simulink model "LFRefMdl"  (R2023b)
settings: Solver=FixedStepDiscrete  StartTime=0.0  StopTime=inf  FixedStep=Ts  RelTol=1e-3
undefined symbols (not defined in the file or in its folder): Cf, Cr, DataType, default_spacing, hasLag, Iz, lf, lr, m, max_ac, max_steer, min_ac, min_steer, NumEgoStates, posSelector, PredictionHorizon, tau, time_gap, Ts, v0_ego
libraries: mpcsigdimcheck_private x19, mpclib x7, simulink x2, mpcadaslib x1, trackingutilitieslib x1, drivinglib x1
(part 1 of 2)
settings Model: Creator=The MathWorks, Inc.  LastModifiedBy=Luca
settings SolverCC: AlgebraicLoopSolver=TrustRegion
settings DataIOCC: SaveOutput=off  SaveTime=off  ReturnWorkspaceOutputs=off
settings OptimizationCC: DefaultParameterBehavior=Inlined  DefaultUnderspecifiedDataType=single  EnhancedBackFolding=on  PassReuseOutputArgsAs=Individual arguments  ZeroExternalMemoryAtStartup=off  ZeroInternalMemoryAtStartup=off  OptimizeBlockOrder=speed  DifferentSizesBufferReuse=on  OptimizationCustomize=off  EfficientTunableParamExpr=on
settings DebuggingCC: ParameterPrecisionLossMsg=none  ParameterTunabilityLossMsg=error  UnconnectedInputMsg=warning  UnconnectedOutputMsg=warning  UnconnectedLineMsg=warning  PregeneratedLibrarySubsystemCodeDiagnostic=none  ArithmeticOperatorsInVariantConditions=warning
settings HardwareCC: ProdLongLongMode=on
settings ModelReferenceCC: EnableRefExpFcnMdlSchedulingChecks=on
settings SFSimCC: SimUseLocalCustomCode=off  MATLABDynamicMemAlloc=off  CustomCodeUndefinedFunction=UseInterfaceOnly  SimTargetLang=C++
settings RTWCC: Description=Embedded Coder  SystemTargetFile=ert.tlc  TemplateMakefile=ert_default_tmf  GenerateReport=on  RTWUseLocalCustomCode=off  BuildConfiguration=Faster Runs  IncludeHyperlinkInReport=on  LaunchReport=on  TargetLang=C++  GenerateTraceInfo=on  GenerateTraceReport=on  GenerateTraceReportSl=on  GenerateTraceReportSf=on  GenerateTraceReportEml=on  DLArmComputeVersion=19.05
settings CodeAppCC: ForceParamTrailComments=on  IgnoreCustomStorageClasses=off  MaxIdLength=63  OperatorAnnotations=on  SimulinkDataObjDesc=on  SFDataObjDesc=on  CustomSymbolStrFcn=$N$M$F  InsertBlockDesc=on
settings ERTTargetCC: TargetLangStandard=C++03 (ISO)  GenerateSampleERTMain=on  CodeInterfacePackaging=C++ class  InlinedParameterPlacement=NonHierarchical  RootIOFormat=Structure reference  ERTCustomFileTemplate=example_file_process.tlc

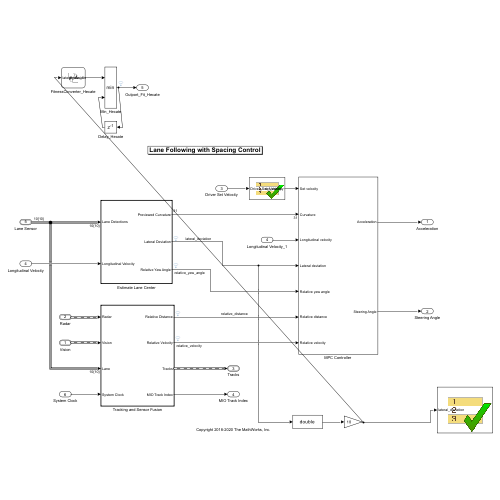
[thumbnail: Simulink's stored preview of the top-level diagram]
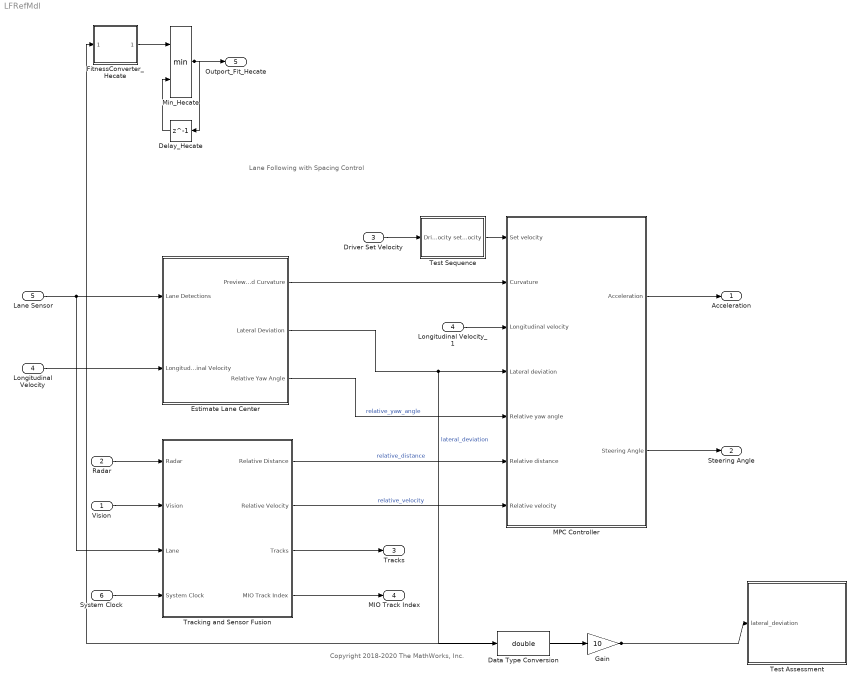
== system LFRefMdl ==
  note: Copyright 2018-2020 The MathWorks, Inc.
  note: Lane Following with Spacing Control
  Vision : Inport  OutDataTypeStr=Bus: BusVision  PortDimensions=[1 1]  BusOutputAsStruct=on
  Radar : Inport  Port=2  OutDataTypeStr=Bus: BusRadar  PortDimensions=[1 1]  BusOutputAsStruct=on
  Driver Set Velocity : Inport  Port=3  OutDataTypeStr=double
  Longitudinal Velocity : Inport  Port=4  OutDataTypeStr=double  Unit=m/s
  Lane Sensor : Inport  Port=5  OutDataTypeStr=Bus: LaneSensor  PortDimensions=[1 1]
  System Clock : Inport  Port=6  OutDataTypeStr=double  PortDimensions=[1 1]
  Data Type Conversion : DataTypeConversion  OutDataTypeStr=double  SaturateOnIntegerOverflow=off  RndMeth=Floor
  Delay_Hecate : Delay  DelayLength=1  InitialCondition=Inf
  Estimate Lane Center : Subsystem  TreatAsAtomicUnit=on  VariantControl=v2
      settings: RTWFileNameOpts=Use function name
  FitnessConverter_Hecate : Stateflow chart  TreatAsAtomicUnit=on
  Gain : Gain  Gain=10
  Longitudinal Velocity_1 : InportShadow  Port=4  OutDataTypeStr=double  Unit=m/s
  "MPC Controller " : Subsystem
  Min_Hecate : MinMax  Inputs=2
  Test Assessment : Test Sequence  TreatAsAtomicUnit=on
  Test Sequence : Test Sequence  TreatAsAtomicUnit=on
  Tracking and Sensor Fusion : Subsystem  TreatAsAtomicUnit=on
      settings: RTWFileNameOpts=Use function name
  Acceleration : Outport  PortDimensions=1  VectorParamsAs1DForOutWhenUnconnected=off
  Steering Angle : Outport  Port=2  PortDimensions=1  VectorParamsAs1DForOutWhenUnconnected=off
  Tracks : Outport  Port=3  OutDataTypeStr=Bus: BusMultiObjectTracker1  PortDimensions=[1 1]  VectorParamsAs1DForOutWhenUnconnected=off  BusOutputAsStruct=on
  MIO Track Index : Outport  Port=4  PortDimensions=1  VectorParamsAs1DForOutWhenUnconnected=off  BusOutputAsStruct=on
  Outport_Fit_Hecate : Outport  Port=5
  wires:
  Longitudinal Velocity/1 -> Estimate Lane Center/2(Longitudinal Velocity)
  Lane Sensor/1 -> Tracking and Sensor Fusion/3(Lane), Estimate Lane Center/1(Lane Detections)
  Vision/1 -> Tracking and Sensor Fusion/2(Vision)
  Radar/1 -> Tracking and Sensor Fusion/1(Radar)
  System Clock/1 -> Tracking and Sensor Fusion/4(System Clock)
  Tracking and Sensor Fusion/3(Tracks) -> Tracks/1
  Tracking and Sensor Fusion/4(MIO Track Index) -> MIO Track Index/1
  Driver Set Velocity/1 -> Test Sequence/1(Driver_Set_Velocity)
  Longitudinal Velocity_1/1 -> "MPC Controller "/3(Longitudinal velocity)
  Estimate Lane Center/1(Previewed Curvature) -> "MPC Controller "/2(Curvature)
  "MPC Controller "/1(Acceleration) -> Acceleration/1
  "MPC Controller "/2(Steering Angle) -> Steering Angle/1
  Estimate Lane Center/2(Lateral Deviation) -> "MPC Controller "/4(Lateral deviation), Data Type Conversion/1  "lateral_deviation"
  Estimate Lane Center/3(Relative Yaw Angle) -> "MPC Controller "/5(Relative yaw angle)  "relative_yaw_angle"
  Tracking and Sensor Fusion/1(Relative Distance) -> "MPC Controller "/6(Relative distance)  "relative_distance"
  Tracking and Sensor Fusion/2(Relative Velocity) -> "MPC Controller "/7(Relative velocity)  "relative_velocity"
  Test Sequence/1(set_velocity) -> "MPC Controller "/1(Set velocity)
  Data Type Conversion/1 -> Gain/1
  Gain/1 -> Test Assessment/1(lateral_deviation), FitnessConverter_Hecate/1(lateral_deviation)
  FitnessConverter_Hecate/1(fitness_1) -> Min_Hecate/1
  Min_Hecate/1 -> Delay_Hecate/1, Outport_Fit_Hecate/1
  Delay_Hecate/1 -> Min_Hecate/2

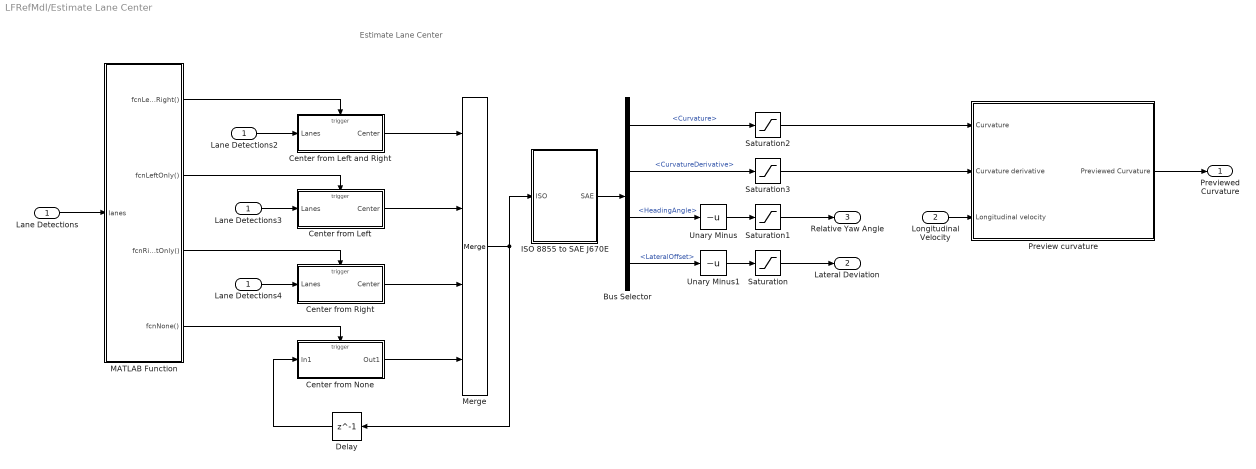
== system LFRefMdl/Estimate Lane Center ==
  note: Estimate Lane Center
  Lane Detections : Inport
  Longitudinal Velocity : Inport  Port=2
  Bus Selector : BusSelector  OutputSignals=Curvature,CurvatureDerivative,HeadingAngle,LateralOffset
  Center from Left : Subsystem  TreatAsAtomicUnit=on
  Center from Left and Right : Subsystem  TreatAsAtomicUnit=on
  Center from None : Subsystem  TreatAsAtomicUnit=on
  Center from Right : Subsystem  TreatAsAtomicUnit=on
  Delay : Delay  DelayLength=1
  ISO 8855 to SAE J670E : Subsystem
  Lane Detections2 : InportShadow
  Lane Detections3 : InportShadow
  Lane Detections4 : InportShadow
  MATLAB Function : MATLAB Function  TreatAsAtomicUnit=on
  Merge : Merge  Inputs=4
  Preview curvature : Subsystem
  Saturation : Saturate  UpperLimit=1.5  LowerLimit=-1.5
  Saturation1 : Saturate  UpperLimit=0.6  LowerLimit=-0.6
  Saturation2 : Saturate  UpperLimit=0.15  LowerLimit=-0.15
  Saturation3 : Saturate  UpperLimit=0.06  LowerLimit=-0.06
  Unary Minus : UnaryMinus
  Unary Minus1 : UnaryMinus
  Previewed Curvature : Outport  VectorParamsAs1DForOutWhenUnconnected=off
  Lateral Deviation : Outport  Port=2  VectorParamsAs1DForOutWhenUnconnected=off
  Relative Yaw Angle : Outport  Port=3  VectorParamsAs1DForOutWhenUnconnected=off
  wires:
  Center from Right/1(Center) -> Merge/3
  Lane Detections3/1 -> Center from Left/1(Lanes)
  Lane Detections4/1 -> Center from Right/1(Lanes)
  MATLAB Function/2(fcnLeftOnly()) -> Center from Left/Trigger
  Center from None/1(Out1) -> Merge/4
  MATLAB Function/1(fcnLeftAndRight()) -> Center from Left and Right/Trigger
  Delay/1 -> Center from None/1(In1)
  Center from Left and Right/1(Center) -> Merge/1
  Lane Detections/1 -> MATLAB Function/1(lanes)
  Lane Detections2/1 -> Center from Left and Right/1(Lanes)
  MATLAB Function/3(fcnRightOnly()) -> Center from Right/Trigger
  MATLAB Function/4(fcnNone()) -> Center from None/Trigger
  Center from Left/1(Center) -> Merge/2
  Merge/1 -> ISO 8855 to SAE J670E/1(ISO), Delay/1
  Saturation3/1 -> Preview curvature/2(Curvature derivative)
  Saturation2/1 -> Preview curvature/1(Curvature)
  Saturation1/1 -> Relative Yaw Angle/1
  Saturation/1 -> Lateral Deviation/1
  Unary Minus/1 -> Saturation1/1
  Preview curvature/1(Previewed Curvature) -> Previewed Curvature/1
  Longitudinal Velocity/1 -> Preview curvature/3(Longitudinal velocity)
  Bus Selector/2 -> Saturation3/1  "<CurvatureDerivative>"
  Bus Selector/1 -> Saturation2/1  "<Curvature>"
  Unary Minus1/1 -> Saturation/1
  Bus Selector/4 -> Unary Minus1/1  "<LateralOffset>"
  Bus Selector/3 -> Unary Minus/1  "<HeadingAngle>"
  ISO 8855 to SAE J670E/1(SAE) -> Bus Selector/1

== system LFRefMdl/MPC Controller  ==
  Set velocity : Inport
  Curvature : Inport  Port=2
  Longitudinal velocity : Inport  Port=3
  Lateral deviation : Inport  Port=4
  Relative yaw angle : Inport  Port=5
  Relative distance : Inport  Port=6
  Relative velocity : Inport  Port=7
  Constant : Constant  Value=time_gap
  Constant1 : Constant  Value=200
  Constant2 : Constant  Value=0
  Path Following Control System : Subsystem  AncestorBlock=mpcadaslib/Path Following Control System  TreatAsAtomicUnit=on  VariantControl=Variant2  mask(Path following control (PFC) system){ModelType=Use vehicle parameters, VehicleMass=m, VehicleYawInertia=Iz, LengthToFront=lf, LengthToRear=lr, FrontTireStiffness=Cf, RearTireStiffness=Cr, AccelTimeConstant=tau, EgoModelMatrixA=[-2,zeros(1,3);1,zeros(1,3);zeros(1,2),-4.4021,-12.4603;zeros(1,2),1.3913,-5.1868], EgoModelMatrixB=[2,zeros(1,3);zeros(1,2),24.1270,15.8609]', EgoModelMatrixC=[zeros(3,1),eye(3)], InitialLongVel=v0_ego, TransportLag=Ts, spaceCtrl=on, DefaultSpacing=default_spacing, MinSteering=min_steer, umin_ext=off, MaxSteering=max_steer, umax_ext=off, MinAcceleration=min_ac, amin_ext=off, MaxAcceleration=max_ac, amax_ext=off, Ts=Ts, PredictionHorizon=PredictionHorizon, ControlHorizon=2, LongWeight=0.1, LateralWeight=1, AccelRateWeight=0.1, SteerRateWeight=0.1, suboptimal=off, maxiter=10, datatypeopt=double, optmode=off, trackmode=off}
      mask prompts: VehicleMass "MPC:adasblocks:promptPFCVehicleMass"; VehicleYawInertia "MPC:adasblocks:promptPFCVehicleInertia"; LengthToFront "MPC:adasblocks:promptPFCVehicleLengthToFront"; LengthToRear "MPC:adasblocks:promptPFCVehicleLengthToRear"; FrontTireStiffness "MPC:adasblocks:promptPFCVehicleFrontStiffness"; RearTireStiffness "MPC:adasblocks:promptPFCVehicleRearStiffness"; AccelTimeConstant "MPC:adasblocks:promptPFCVehicleTimeConstant"; EgoModelMatrixA "MPC:adasblocks:promptPFCMatrixA"; EgoModelMatrixB "MPC:adasblocks:promptPFCMatrixB"; EgoModelMatrixC "MPC:adasblocks:promptPFCMatrixC"; InitialLongVel "MPC:adasblocks:promptPFCInitialLongitudinalVelocity"; TransportLag "MPC:adasblocks:promptPFCTransportLag"; spaceCtrl "MPC:adasblocks:promptPFCSpacingControl"; DefaultSpacing "MPC:adasblocks:promptPFCDefaultSpacing"; MinSteering "MPC:adasblocks:promptPFCMinSteering"; umin_ext "MPC:adasblocks:promptPFCUseExternalSource"; MaxSteering "MPC:adasblocks:promptPFCMaxSteering"; umax_ext "MPC:adasblocks:promptPFCUseExternalSource"; MinAcceleration "MPC:adasblocks:promptPFCMinAcceleration"; amin_ext "MPC:adasblocks:promptPFCUseExternalSource"; MaxAcceleration "MPC:adasblocks:promptPFCMaxAcceleration"; amax_ext "MPC:adasblocks:promptPFCUseExternalSource"; Ts "MPC:adasblocks:promptPFCSampleTime"; PredictionHorizon "MPC:adasblocks:promptPFCPredictionSteps"; ControlHorizon "MPC:adasblocks:promptPFCControlHorizon"; LongWeight "MPC:adasblocks:promptPFCLongWeight"; LateralWeight "MPC:adasblocks:promptPFCLateralWeight"; AccelRateWeight "MPC:adasblocks:promptPFCAccelRateWeight"; SteerRateWeight "MPC:adasblocks:promptPFCSteerRateWeight"; suboptimal "MPC:adasblocks:promptPFCUseSubOptimal"; maxiter "MPC:adasblocks:promptPFCMaxIter"; datatypeopt "MPC:adasblocks:promptPFCDataType"; optmode "MPC:adasblocks:promptPFCMPCOptimize"; trackmode "MPC:adasblocks:promptPFCSmoothTransition"
      mask help: MPC:adasblocks:pfcMaskDescription
      mask init:
      | [mpcobj,hasSpacingCtrl,UseExternalModel,DataType,NumEgoStates,hasLag] = ...
      |     pfcblock_MaskInitFcn(gcb,EgoModelMatrixA,EgoModelMatrixB,EgoModelMatrixC,...
      |     MaxSteering,MinSteering,...
      |     MaxAcceleration,MinAcceleration,...
      |     InitialLongVel,DefaultSpacing,...
      |     PredictionHorizon,ControlHorizon,Ts,maxiter,AccelRateWeight,SteerRateWeight,LongWeight,LateralWeight,...
      |     VehicleMass,VehicleYawInertia,LengthToFront,LengthToRear,FrontTireStiffness,RearTireStiffness,TransportLag,AccelTimeConstant);
      settings: RTWFileNameOpts=Use function name
      mask Help: eval('mpcCSHelp(''mpcBlockPFC'')');
      mask TypeOptions ModelType: MPC:adasblocks:promptPFCUseVehicleParameters | MPC:adasblocks:promptPFCUseVehicleModel
      mask Callback ModelType: pfcblock_callbackModelType(gcb);
      mask Callback spaceCtrl: pfcblock_callbackSpacingCtrl(gcb);
      mask Callback umin_ext: adasblocks_utilUseExternal(gcb,'MinSteering','umin_ext');
      mask Callback umax_ext: adasblocks_utilUseExternal(gcb,'MaxSteering','umax_ext');
      mask Callback amin_ext: adasblocks_utilUseExternal(gcb,'MinAcceleration','amin_ext');
      mask Callback amax_ext: adasblocks_utilUseExternal(gcb,'MaxAcceleration','amax_ext');
      mask Callback suboptimal: adasblocks_callbackUsesuboptimal(gcb);
      mask TypeOptions datatypeopt: double | single
      mask DialogControl DescTextVar Tooltip: MPC:adasblocks:ttipPFCMaskDescription
      mask DialogControl Container4 Prompt: MPC:adasblocks:promptPFCTabParameters
      mask DialogControl Container11 Prompt: MPC:adasblocks:promptPFCEgoVehicle
      mask DialogControl Control4 Prompt: MPC:adasblocks:promptPFCLinearModel
      mask DialogControl ModelType Tooltip: MPC:adasblocks:ttipPFCModelDynamics
      mask DialogControl UseParam Prompt: MPC:adasblocks:promptPFCSpecifyVehicleParameters
      mask DialogControl VehicleMass Prompt: Total mass (kg)
      mask DialogControl VehicleMass Tooltip: MPC:adasblocks:ttipPFCVehicleMass
      mask DialogControl VehicleYawInertia Prompt: Yaw moment of inertia (kgm^2)
      mask DialogControl VehicleYawInertia Tooltip: MPC:adasblocks:ttipPFCVehicleInertia
      mask DialogControl LengthToFront Prompt: Longitudinal distance from center of gravity to front tires (m)
      mask DialogControl LengthToFront Tooltip: MPC:adasblocks:ttipPFCVehicleLengthToFront
      mask DialogControl LengthToRear Prompt: Longitudinal distance from center of gravity to rear tires (m)
      mask DialogControl LengthToRear Tooltip: MPC:adasblocks:ttipPFCVehicleLengthToRear
      mask DialogControl FrontTireStiffness Prompt: Cornering stiffness of front tires (N/rad)
      mask DialogControl FrontTireStiffness Tooltip: MPC:adasblocks:ttipPFCVehicleFrontStiffness
      mask DialogControl RearTireStiffness Prompt: Cornering stiffness of rear tires (N/rad)
      mask DialogControl RearTireStiffness Tooltip: MPC:adasblocks:ttipPFCVehicleRearStiffness
      mask DialogControl AccelTimeConstant Prompt: Longitudinal acceleration tracking time constant (s)
      mask DialogControl AccelTimeConstant Tooltip: MPC:adasblocks:ttipPFCAccelTimeConstant
      mask DialogControl UseModel Prompt: MPC:adasblocks:promptPFCSpecifyVehicleModel
      mask DialogControl EgoModelMatrixA Prompt: A
      mask DialogControl EgoModelMatrixA Tooltip: MPC:adasblocks:ttipPFCEgoModelMatrixA
      mask DialogControl EgoModelMatrixB Prompt: B
      mask DialogControl EgoModelMatrixB Tooltip: MPC:adasblocks:ttipPFCEgoModelMatrixB
      mask DialogControl EgoModelMatrixC Prompt: C
      mask DialogControl EgoModelMatrixC Tooltip: MPC:adasblocks:ttipPFCEgoModelMatrixC
      mask DialogControl InitialLongVel Prompt: Initial longitudinal velocity (m/s)
      mask DialogControl InitialLongVel Tooltip: MPC:adasblocks:ttipPFCInitialLongVelocity
      mask DialogControl TransportLag Prompt: Transport lag between model inputs and outputs (s)
      mask DialogControl TransportLag Tooltip: MPC:adasblocks:ttipPFCTransportLag
      mask DialogControl Container25 Prompt: MPC:adasblocks:promptPFCSpacingCtrl
      mask DialogControl spaceCtrl Prompt: Maintain safe distance between lead vehicle and ego vehicle
      mask DialogControl spaceCtrl Tooltip: MPC:adasblocks:ttipPFCEnableSpacingCtrl
      mask DialogControl DefaultSpacing Prompt: Default spacing (m)
      mask DialogControl DefaultSpacing Tooltip: MPC:adasblocks:ttipPFCDefaultSpacing
      mask DialogControl Container21 Prompt: MPC:adasblocks:promptPFCTabController
      mask DialogControl Container12 Prompt: MPC:adasblocks:promptPFCConstraints
      mask DialogControl MinSteering Prompt: Minimum steering angle (rad)
      mask DialogControl MinSteering Tooltip: MPC:adasblocks:ttipPFCMinSteering
      mask DialogControl umin_ext Prompt: Use external source
      mask DialogControl MaxSteering Prompt: Maximum steering angle (rad)
      mask DialogControl MaxSteering Tooltip: MPC:adasblocks:ttipPFCMaxSteering
      mask DialogControl umax_ext Prompt: Use external source
      mask DialogControl MinAcceleration Prompt: Minimum longitudinal acceleration (m/s^2)
      mask DialogControl MinAcceleration Tooltip: MPC:adasblocks:ttipPFCMaxDeceleration
      mask DialogControl amin_ext Prompt: Use external source
      mask DialogControl MaxAcceleration Prompt: Maximum longitudinal acceleration (m/s^2)
      mask DialogControl MaxAcceleration Tooltip: MPC:adasblocks:ttipPFCMaxAcceleration
      mask DialogControl amax_ext Prompt: Use external source
      mask DialogControl Container15 Prompt: MPC:adasblocks:promptPFCMPCSettings
      mask DialogControl Ts Prompt: Sample time (s)
      mask DialogControl Ts Tooltip: MPC:adasblocks:ttipPFCSampleTime
      mask DialogControl PredictionHorizon Prompt: Prediction horizon (steps)
      mask DialogControl PredictionHorizon Tooltip: MPC:adasblocks:ttipPFCPredictionSteps
      mask DialogControl ControlHorizon Prompt: Control horizon (steps)
      mask DialogControl ControlHorizon Tooltip: MPC:adasblocks:ttipPFCControlHorizon
      mask DialogControl Container18 Prompt: MPC:adasblocks:promptPFCWeight
      mask DialogControl LongWeight Prompt: Weight on velocity tracking
      mask DialogControl LongWeight Tooltip: MPC:adasblocks:ttipPFCLongWeight
      mask DialogControl LateralWeight Prompt: Weight on lateral error
      mask DialogControl LateralWeight Tooltip: MPC:adasblocks:ttipPFCLateralWeight
      mask DialogControl AccelRateWeight Prompt: Weight on change of longitudinal acceleration
      mask DialogControl AccelRateWeight Tooltip: MPC:adasblocks:ttipPFCAccelRateWeight
      mask DialogControl SteerRateWeight Prompt: Weight on change of steering angle
      mask DialogControl SteerRateWeight Tooltip: MPC:adasblocks:ttipPFCSteerRateWeight
      mask DialogControl Container6 Prompt: MPC:adasblocks:promptPFCTabBlock
      mask DialogControl Container7 Prompt: MPC:adasblocks:promptPFCOptimization
      mask DialogControl suboptimal Prompt: Use suboptimal solution
      mask DialogControl suboptimal Tooltip: MPC:adasblocks:ttipPFCUseSubOptimal
      mask DialogControl maxiter Prompt: Maximum iteration number
      mask DialogControl maxiter Tooltip: MPC:adasblocks:ttipPFCMaxIter
      mask DialogControl datatypeopt Prompt: Data Type
      mask DialogControl datatypeopt Tooltip: MPC:adasblocks:ttipPFCDataType
      mask DialogControl Container9 Prompt: MPC:adasblocks:promptPFCBlockOptions
      mask DialogControl optmode Prompt: Use external signal to enable or disable optimization
      mask DialogControl optmode Tooltip: MPC:adasblocks:ttipPFCMPCOptimize
      mask DialogControl trackmode Prompt: Use external control signal for bumpless transfer between PFC and other controllers
      mask DialogControl trackmode Tooltip: MPC:adasblocks:ttipPFCSmoothTransition
      mask DialogControl Container10 Prompt: MPC:adasblocks:promptPFCCustomizeText
      mask DialogControl Control2 Prompt: MPC:adasblocks:promptPFCCreateSystemTextMore
      mask DialogControl Control3 Prompt: MPC:adasblocks:promptPFCCreateSysBtn
      mask DialogControl Control3 Tooltip: MPC:adasblocks:ttipPFCCreateSysBtn
      mask DialogControl Control3 Callback: pfcblock_callbackCreateSubsystemButton(gcb);
  Switch1 : Switch  Criteria=u2 > Threshold  Threshold=1000  SaturateOnIntegerOverflow=off  InputSameDT=off
  Switch2 : Switch  Criteria=u2 > Threshold  Threshold=1000  SaturateOnIntegerOverflow=off  InputSameDT=off
  Acceleration : Outport  VectorParamsAs1DForOutWhenUnconnected=off
  Steering Angle : Outport  Port=2  VectorParamsAs1DForOutWhenUnconnected=off
  wires:
  Path Following Control System/1(Longitudinal acceleration) -> Acceleration/1
  Path Following Control System/2(Steering angle) -> Steering Angle/1
  Set velocity/1 -> Path Following Control System/1(Set velocity)
  Curvature/1 -> Path Following Control System/6(Curvature)
  Longitudinal velocity/1 -> Path Following Control System/5(Longitudinal velocity)
  Lateral deviation/1 -> Path Following Control System/7(Lateral deviation)
  Relative yaw angle/1 -> Path Following Control System/8(Relative yaw angle)
  Relative distance/1 -> Switch2/2, Switch1/3, Switch1/2
  Constant1/1 -> Switch1/1
  Relative velocity/1 -> Switch2/3
  Constant2/1 -> Switch2/1
  Constant/1 -> Path Following Control System/2(Time gap)
  Switch1/1 -> Path Following Control System/3(Relative distance)
  Switch2/1 -> Path Following Control System/4(Relative velocity)

== system LFRefMdl/Tracking and Sensor Fusion ==
  note: Tracking and Sensor Fusion
  note: Sensor Fusion
  Radar : Inport  OutDataTypeStr=Bus: BusRadar  PortDimensions=[1 1]  BusOutputAsStruct=on
  Vision : Inport  Port=2  OutDataTypeStr=Bus: BusVision  PortDimensions=[1 1]  BusOutputAsStruct=on
  Lane : Inport  Port=3  OutDataTypeStr=Bus: LaneSensor  BusOutputAsStruct=on
  System Clock : Inport  Port=4  OutDataTypeStr=double  PortDimensions=[1 1]
  Detection Concatenation1 : trackingutilitieslib/Detection Concatenation  NumInputs=2  BusNameSource=Auto  BusName=BusDetectionConcatenation1  SimulateUsing=Interpreted execution
  Find Lead Car : MATLAB Function  TreatAsAtomicUnit=on
  Multi-Object Tracker : drivinglib/Multi-Object Tracker  TrackerIndex=uint32( 0 )  FilterInitializationFcn=initcvekf  AssignmentThreshold=assigThresh  ConfirmationThreshold=[ 2, 3 ]  DeletionThreshold=[ 5, 5 ]  MaxNumTracks=numTracks  MaxNumSensors=numSensors  OOSMHandling=Terminate  StateParametersSimulink=struct  HasStateParametersInput=off  TimeInputSource=Input port  HasCostMatrixInput=off  HasDetectableTrackIDsInput=off  BusNameSource=Property  BusName=BusMultiObjectTracker1  TentativeTracksOutputPort=off  AllTracksOutputPort=off  SimulateUsing=Interpreted execution
  Position Selector : Constant  Value=posSelector
  Relative Distance : Outport  VectorParamsAs1DForOutWhenUnconnected=off
  Relative Velocity : Outport  Port=2  VectorParamsAs1DForOutWhenUnconnected=off
  Tracks : Outport  Port=3  OutDataTypeStr=Bus:BusMultiObjectTracker1  PortDimensions=[1 1]  VectorParamsAs1DForOutWhenUnconnected=off  BusOutputAsStruct=on
  MIO Track Index : Outport  Port=4  VectorParamsAs1DForOutWhenUnconnected=off
  wires:
  Find Lead Car/2(vx) -> Relative Velocity/1
  Find Lead Car/3(mioTrackIndex) -> MIO Track Index/1
  Find Lead Car/1(x) -> Relative Distance/1
  Position Selector/1 -> Find Lead Car/3(positionSelector)
  Lane/1 -> Find Lead Car/2(lane)
  Detection Concatenation1/1 -> Multi-Object Tracker/1
  Multi-Object Tracker/1 -> Find Lead Car/1(confirmedTracks), Tracks/1
  System Clock/1 -> Multi-Object Tracker/2
  Vision/1 -> Detection Concatenation1/1
  Radar/1 -> Detection Concatenation1/2

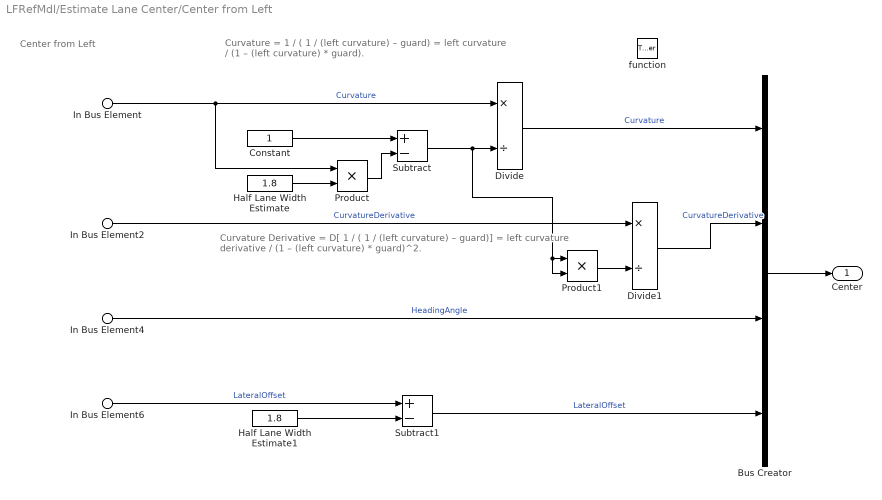
== system LFRefMdl/Estimate Lane Center/Center from Left ==
  note: Curvature Derivative
      | = D[ 1 / ( 1 / (left curvature) – guard)]
      | = left curvature derivative / (1 – (left curvature) * guard)^2.
  note: Center from Left
  note: Curvature
      | = 1 / ( 1 / (left curvature) – guard)
      | = left curvature / (1 – (left curvature) * guard).
  In Bus Element : Inport  PortName=Lanes  Element=Left.Curvature
  In Bus Element2 : Inport  PortName=Lanes  Element=Left.CurvatureDerivative
  In Bus Element4 : Inport  PortName=Lanes  Element=Left.HeadingAngle
  In Bus Element6 : Inport  PortName=Lanes  Element=Left.LateralOffset
  function : TriggerPort  TriggerType=function-call  VariantControl=Variant
  Bus Creator : BusCreator  Inputs=4
  Constant : Constant  OutDataTypeStr=Inherit: Inherit via back propagation
  Divide : Product  Inputs=*/
  Divide1 : Product  Inputs=*/
  Half Lane Width Estimate : Constant  Value=1.8  OutDataTypeStr=Inherit: Inherit via back propagation
  Half Lane Width Estimate1 : Constant  Value=1.8  OutDataTypeStr=Inherit: Inherit via back propagation
  Product : Product
  Product1 : Product
  Subtract : Sum  Inputs=+-
  Subtract1 : Sum  Inputs=+-
  Center : Outport  VectorParamsAs1DForOutWhenUnconnected=off
  wires:
  Product/1 -> Subtract/2
  Half Lane Width Estimate1/1 -> Subtract1/2
  In Bus Element6/1 -> Subtract1/1  "LateralOffset"
  Product1/1 -> Divide1/2
  In Bus Element2/1 -> Divide1/1  "CurvatureDerivative"
  Constant/1 -> Subtract/1
  Half Lane Width Estimate/1 -> Product/2
  Subtract/1 -> Divide/2, Product1/1, Product1/2
  In Bus Element/1 -> Divide/1, Product/1  "Curvature"
  Subtract1/1 -> Bus Creator/4  "LateralOffset"
  In Bus Element4/1 -> Bus Creator/3  "HeadingAngle"
  Divide/1 -> Bus Creator/1  "Curvature"
  Divide1/1 -> Bus Creator/2  "CurvatureDerivative"
  Bus Creator/1 -> Center/1

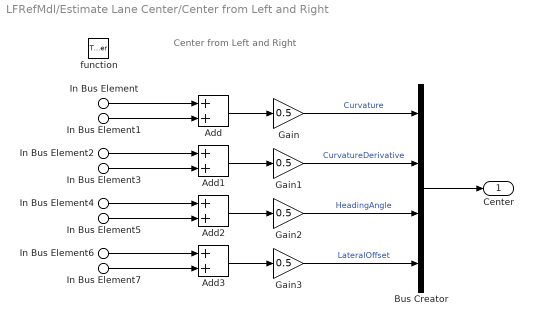
== system LFRefMdl/Estimate Lane Center/Center from Left and Right ==
  note: Center from Left and Right
  In Bus Element : Inport  PortName=Lanes  Element=Left.Curvature
  In Bus Element2 : Inport  PortName=Lanes  Element=Left.CurvatureDerivative
  In Bus Element4 : Inport  PortName=Lanes  Element=Left.HeadingAngle
  In Bus Element6 : Inport  PortName=Lanes  Element=Left.LateralOffset
  In Bus Element1 : Inport  PortName=Lanes  Element=Right.Curvature
  In Bus Element3 : Inport  PortName=Lanes  Element=Right.CurvatureDerivative
  In Bus Element5 : Inport  PortName=Lanes  Element=Right.HeadingAngle
  In Bus Element7 : Inport  PortName=Lanes  Element=Right.LateralOffset
  function : TriggerPort  TriggerType=function-call  VariantControl=Variant
  Add{,1..3} (4 alike) : Sum
  Bus Creator : BusCreator  Inputs=4
  Gain{,1..3} (4 alike) : Gain  Gain=0.5
  Center : Outport  VectorParamsAs1DForOutWhenUnconnected=off
  wires:
  In Bus Element6/1 -> Add3/1
  In Bus Element7/1 -> Add3/2
  In Bus Element5/1 -> Add2/2
  In Bus Element4/1 -> Add2/1
  In Bus Element3/1 -> Add1/2
  In Bus Element2/1 -> Add1/1
  In Bus Element1/1 -> Add/2
  In Bus Element/1 -> Add/1
  Bus Creator/1 -> Center/1
  Gain3/1 -> Bus Creator/4  "LateralOffset"
  Add3/1 -> Gain3/1
  Gain2/1 -> Bus Creator/3  "HeadingAngle"
  Add2/1 -> Gain2/1
  Gain1/1 -> Bus Creator/2  "CurvatureDerivative"
  Add1/1 -> Gain1/1
  Gain/1 -> Bus Creator/1  "Curvature"
  Add/1 -> Gain/1

== system LFRefMdl/Estimate Lane Center/Center from None ==
  In1 : Inport
  function : TriggerPort  TriggerType=function-call  VariantControl=Variant
  Out1 : Outport  VectorParamsAs1DForOutWhenUnconnected=off
  wires:
  In1/1 -> Out1/1

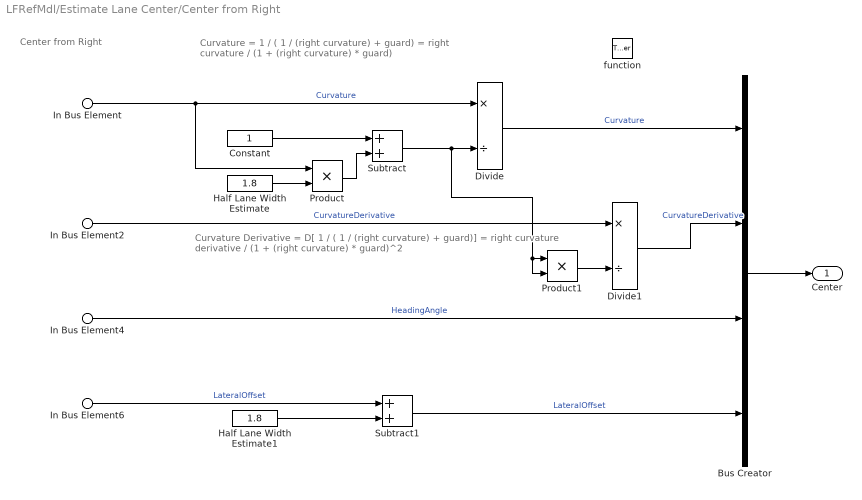
== system LFRefMdl/Estimate Lane Center/Center from Right ==
  note: Curvature Derivative
      | = D[ 1 / ( 1 / (right curvature) + guard)]
      | = right curvature derivative / (1 + (right curvature) * guard)^2
  note: Curvature
      | = 1 / ( 1 / (right curvature) + guard)
      | = right curvature / (1 + (right curvature) * guard)
  note: Center from Right
  In Bus Element : Inport  PortName=Lanes  Element=Right.Curvature
  In Bus Element2 : Inport  PortName=Lanes  Element=Right.CurvatureDerivative
  In Bus Element4 : Inport  PortName=Lanes  Element=Right.HeadingAngle
  In Bus Element6 : Inport  PortName=Lanes  Element=Right.LateralOffset
  function : TriggerPort  TriggerType=function-call  VariantControl=Variant
  Bus Creator : BusCreator  Inputs=4
  Constant : Constant  OutDataTypeStr=Inherit: Inherit via back propagation
  Divide : Product  Inputs=*/
  Divide1 : Product  Inputs=*/
  Half Lane Width Estimate : Constant  Value=1.8  OutDataTypeStr=Inherit: Inherit via back propagation
  Half Lane Width Estimate1 : Constant  Value=1.8  OutDataTypeStr=Inherit: Inherit via back propagation
  Product : Product
  Product1 : Product
  Subtract : Sum
  Subtract1 : Sum
  Center : Outport  VectorParamsAs1DForOutWhenUnconnected=off
  wires:
  Half Lane Width Estimate/1 -> Product/2
  Product/1 -> Subtract/2
  Constant/1 -> Subtract/1
  Subtract/1 -> Divide/2, Product1/1, Product1/2
  In Bus Element/1 -> Divide/1, Product/1  "Curvature"
  Bus Creator/1 -> Center/1
  Subtract1/1 -> Bus Creator/4  "LateralOffset"
  Divide/1 -> Bus Creator/1  "Curvature"
  In Bus Element6/1 -> Subtract1/1  "LateralOffset"
  Half Lane Width Estimate1/1 -> Subtract1/2
  In Bus Element4/1 -> Bus Creator/3  "HeadingAngle"
  Product1/1 -> Divide1/2
  Divide1/1 -> Bus Creator/2  "CurvatureDerivative"
  In Bus Element2/1 -> Divide1/1  "CurvatureDerivative"

== system LFRefMdl/Estimate Lane Center/ISO 8855 to SAE J670E ==
  note: positive Y is to the left in ISO 8855
      | positive Y is to the right in SAE J670E
  note: ISO 8855 to SAE J670E
  ISO : Inport
  Bus Creator : BusCreator  Inputs=4
  Bus Selector : BusSelector  OutputSignals=CurvatureDerivative,Curvature,HeadingAngle,LateralOffset
  Signal Specification : SignalSpecification  Unit=1/m^2
  Signal Specification1 : SignalSpecification  Unit=1/m
  Signal Specification2 : SignalSpecification  Unit=rad
  Signal Specification3 : SignalSpecification  Unit=m
  Unary Minus{,1..3} (4 alike) : UnaryMinus
  SAE : Outport  VectorParamsAs1DForOutWhenUnconnected=off
  wires:
  ISO/1 -> Bus Selector/1
  Bus Selector/2 -> Unary Minus/1  "<Curvature>"
  Bus Selector/1 -> Unary Minus1/1  "<CurvatureDerivative>"
  Bus Selector/3 -> Unary Minus2/1  "<HeadingAngle>"
  Bus Selector/4 -> Unary Minus3/1  "<LateralOffset>"
  Bus Creator/1 -> SAE/1
  Signal Specification/1 -> Bus Creator/2  "Curvature"
  Unary Minus1/1 -> Signal Specification1/1
  Unary Minus2/1 -> Signal Specification2/1
  Unary Minus3/1 -> Signal Specification3/1
  Unary Minus/1 -> Signal Specification/1
  Signal Specification1/1 -> Bus Creator/1  "CurvatureDerivative"
  Signal Specification2/1 -> Bus Creator/3  "HeadingAngle"
  Signal Specification3/1 -> Bus Creator/4  "LateralOffset"

== system LFRefMdl/Estimate Lane Center/Preview curvature ==
  Curvature : Inport
  Curvature derivative : Inport  Port=2
  Longitudinal velocity : Inport  Port=3
  Gain : Gain  Gain=[0:Ts:PredictionHorizon*Ts]'
  Gain1 : Gain
  Product : Product
  Sum : Sum
  Previewed Curvature : Outport  VectorParamsAs1DForOutWhenUnconnected=off
  wires:
  Sum/1 -> Previewed Curvature/1
  Curvature/1 -> Gain1/1
  Gain/1 -> Sum/2
  Product/1 -> Gain/1
  Longitudinal velocity/1 -> Product/2
  Curvature derivative/1 -> Product/1
  Gain1/1 -> Sum/1

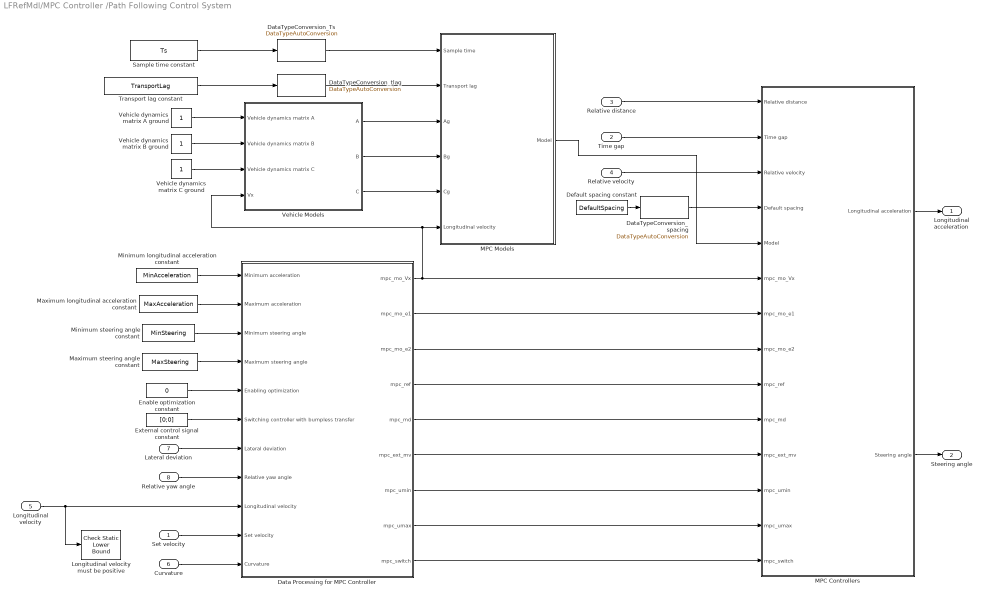
== system LFRefMdl/MPC Controller /Path Following Control System ==
  Set velocity : Inport
  Time gap : Inport  Port=2
  Relative distance : Inport  Port=3
  Relative velocity : Inport  Port=4
  Longitudinal velocity : Inport  Port=5
  Curvature : Inport  Port=6
  Lateral deviation : Inport  Port=7
  Relative yaw angle : Inport  Port=8
  Data Processing for MPC Controller : Subsystem
  DataTypeConversion_Ts : mpcsigdimcheck_private/DataTypeAutoConversion  datatypestr=DataType
  DataTypeConversion_spacing : mpcsigdimcheck_private/DataTypeAutoConversion  datatypestr=DataType
  DataTypeConversion_tlag : mpcsigdimcheck_private/DataTypeAutoConversion  datatypestr=DataType
  Default spacing constant : Constant  Value=DefaultSpacing
  Enable optimization constant : Constant  Value=0
  External control signal constant : Constant  Value=[0;0]  VectorParams1D=off
  Longitudinal velocity must be positive : simulink/Model Verification/Check Static  Lower Bound  Description=0 < u  min=0  min_included=off  enabled=on  stopWhenAssertionFail=off  export=off  icon=graphic
  MPC Controllers : Subsystem  Variant=on  VariantControlMode=label  VariantControl=Variant1  LabelModeActiveChoice=pathFollowingHasSpacingCtrl
  MPC Models : Subsystem  Variant=on  VariantControlMode=label  VariantControl=Variant1  LabelModeActiveChoice=pathFollowingHasSpacingCtrl
  Maximum longitudinal acceleration constant : Constant  Value=MaxAcceleration
  Maximum steering angle constant : Constant  Value=MaxSteering
  Minimum longitudinal acceleration constant : Constant  Value=MinAcceleration
  Minimum steering angle constant : Constant  Value=MinSteering
  Sample time constant : Constant  Value=Ts
  Transport lag constant : Constant  Value=TransportLag
  Vehicle Models : Subsystem  Variant=on  VariantControlMode=label  VariantControl=Variant1  LabelModeActiveChoice=useVehicleParameters
  Vehicle dynamics matrix A ground : Constant
  Vehicle dynamics matrix B ground : Constant
  Vehicle dynamics matrix C ground : Constant
  Longitudinal acceleration : Outport  PortDimensions=1  VectorParamsAs1DForOutWhenUnconnected=off
  Steering angle : Outport  Port=2  VectorParamsAs1DForOutWhenUnconnected=off
  wires:
  DataTypeConversion_spacing/1 -> MPC Controllers/4("Default spacing ")
  DataTypeConversion_tlag/1 -> MPC Models/2(Transport lag)
  DataTypeConversion_Ts/1 -> MPC Models/1(Sample time)
  Vehicle dynamics matrix B ground/1 -> Vehicle Models/2(Vehicle dynamics matrix B)
  Vehicle dynamics matrix C ground/1 -> Vehicle Models/3(Vehicle dynamics matrix C)
  Vehicle dynamics matrix A ground/1 -> Vehicle Models/1(Vehicle dynamics matrix A)
  Sample time constant/1 -> DataTypeConversion_Ts/1
  Transport lag constant/1 -> DataTypeConversion_tlag/1
  Vehicle Models/3(" C") -> MPC Models/5(Cg)
  Vehicle Models/2(" B") -> MPC Models/4(Bg)
  Vehicle Models/1(" A") -> MPC Models/3(Ag)
  Minimum steering angle constant/1 -> Data Processing for MPC Controller/3(Minimum steering angle)
  Minimum longitudinal acceleration constant/1 -> Data Processing for MPC Controller/1(Minimum acceleration)
  External control signal constant/1 -> Data Processing for MPC Controller/6(Switching controller with bumpless transfer)
  Enable optimization constant/1 -> Data Processing for MPC Controller/5(Enabling optimization)
  Maximum steering angle constant/1 -> Data Processing for MPC Controller/4(Maximum steering angle)
  Maximum longitudinal acceleration constant/1 -> Data Processing for MPC Controller/2(Maximum acceleration)
  Relative yaw angle/1 -> Data Processing for MPC Controller/8(Relative yaw angle)
  Lateral deviation/1 -> Data Processing for MPC Controller/7(Lateral deviation)
  Set velocity/1 -> Data Processing for MPC Controller/10(Set velocity)
  Curvature/1 -> Data Processing for MPC Controller/11(Curvature)
  Data Processing for MPC Controller/7(mpc_umin) -> MPC Controllers/12("mpc_umin ")
  Data Processing for MPC Controller/6(mpc_ext_mv) -> MPC Controllers/11("mpc_ext_mv ")
  Data Processing for MPC Controller/2(mpc_mo_e1) -> MPC Controllers/7("mpc_mo_e1 ")
  Longitudinal velocity/1 -> Longitudinal velocity must be positive/1, Data Processing for MPC Controller/9(Longitudinal velocity)
  Data Processing for MPC Controller/4(mpc_ref) -> MPC Controllers/9("mpc_ref ")
  Data Processing for MPC Controller/3(mpc_mo_e2) -> MPC Controllers/8("mpc_mo_e2 ")
  Data Processing for MPC Controller/5(mpc_md) -> MPC Controllers/10("mpc_md ")
  Data Processing for MPC Controller/1(mpc_mo_Vx) -> Vehicle Models/4("Vx "), MPC Models/6("Longitudinal velocity "), MPC Controllers/6("mpc_mo_Vx ")
  MPC Controllers/2("  Steering angle") -> Steering angle/1
  Data Processing for MPC Controller/8(mpc_umax) -> MPC Controllers/13("mpc_umax ")
  MPC Models/1(" Model") -> MPC Controllers/5("Model ")
  Data Processing for MPC Controller/9(mpc_switch) -> MPC Controllers/14("mpc_switch ")
  Default spacing constant/1 -> DataTypeConversion_spacing/1
  MPC Controllers/1(" Longitudinal acceleration") -> Longitudinal acceleration/1
  Time gap/1 -> MPC Controllers/2("Time gap ")
  Relative distance/1 -> MPC Controllers/1("Relative distance ")
  Relative velocity/1 -> MPC Controllers/3("Relative velocity ")

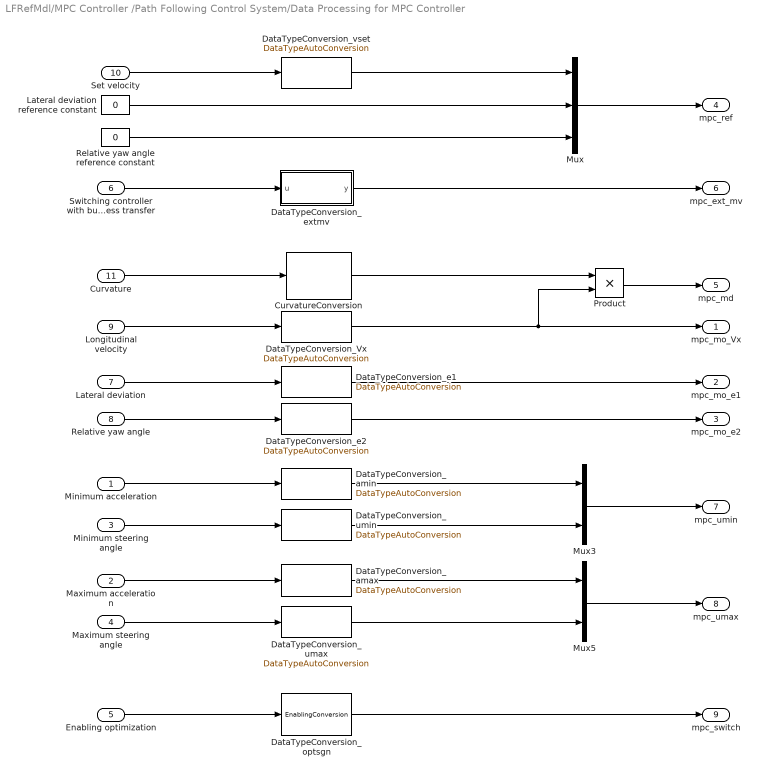
== system LFRefMdl/MPC Controller /Path Following Control System/Data Processing for MPC Controller ==
  Minimum acceleration : Inport
  Maximum acceleration : Inport  Port=2
  Minimum steering angle : Inport  Port=3
  Maximum steering angle : Inport  Port=4
  Enabling optimization : Inport  Port=5
  Switching controller with bumpless transfer : Inport  Port=6
  Lateral deviation : Inport  Port=7
  Relative yaw angle : Inport  Port=8
  Longitudinal velocity : Inport  Port=9
  Set velocity : Inport  Port=10
  Curvature : Inport  Port=11
  CurvatureConversion : mpcsigdimcheck_private/CurvatureConversion  datatypestr=DataType  p=PredictionHorizon
  DataTypeConversion_Vx : mpcsigdimcheck_private/DataTypeAutoConversion  datatypestr=DataType
  DataTypeConversion_amax : mpcsigdimcheck_private/DataTypeAutoConversion  datatypestr=DataType
  DataTypeConversion_amin : mpcsigdimcheck_private/DataTypeAutoConversion  datatypestr=DataType
  DataTypeConversion_e1 : mpcsigdimcheck_private/DataTypeAutoConversion  datatypestr=DataType
  DataTypeConversion_e2 : mpcsigdimcheck_private/DataTypeAutoConversion  datatypestr=DataType
  DataTypeConversion_extmv : MATLAB Function  TreatAsAtomicUnit=on  mask(MPCDataTypeAutoConversion){datatypestr=DataType}
      mask prompts: datatypestr "Data type"
      mask init:
      | isDouble = strcmp(datatypestr,'double');
  DataTypeConversion_optsgn : mpcsigdimcheck_private/EnablingConversion  SystemSampleTime=-1  VariantActivationTime=update diagram  AllowFlexibleInterface=on  Latency=0  AutoFrameSizeCalculation=off
  DataTypeConversion_umax : mpcsigdimcheck_private/DataTypeAutoConversion  datatypestr=DataType
  DataTypeConversion_umin : mpcsigdimcheck_private/DataTypeAutoConversion  datatypestr=DataType
  DataTypeConversion_vset : mpcsigdimcheck_private/DataTypeAutoConversion  datatypestr=DataType
  Lateral deviation reference constant : Constant  Value=0  OutDataTypeStr=DataType
  Mux : Mux  Inputs=3
  Mux3 : Mux  Inputs=2
  Mux5 : Mux  Inputs=2
  Product : Product
  "Relative yaw angle reference constant " : Constant  Value=0  OutDataTypeStr=DataType
  mpc_mo_Vx : Outport  VectorParamsAs1DForOutWhenUnconnected=off
  mpc_mo_e1 : Outport  Port=2  VectorParamsAs1DForOutWhenUnconnected=off
  mpc_mo_e2 : Outport  Port=3  VectorParamsAs1DForOutWhenUnconnected=off
  mpc_ref : Outport  Port=4  VectorParamsAs1DForOutWhenUnconnected=off
  mpc_md : Outport  Port=5  VectorParamsAs1DForOutWhenUnconnected=off
  mpc_ext_mv : Outport  Port=6  VectorParamsAs1DForOutWhenUnconnected=off
  mpc_umin : Outport  Port=7  VectorParamsAs1DForOutWhenUnconnected=off
  mpc_umax : Outport  Port=8  VectorParamsAs1DForOutWhenUnconnected=off
  mpc_switch : Outport  Port=9  VectorParamsAs1DForOutWhenUnconnected=off
  wires:
  DataTypeConversion_optsgn/1 -> mpc_switch/1
  Enabling optimization/1 -> DataTypeConversion_optsgn/1
  DataTypeConversion_e1/1 -> mpc_mo_e1/1
  Mux/1 -> mpc_ref/1
  DataTypeConversion_vset/1 -> Mux/1
  Relative yaw angle/1 -> DataTypeConversion_e2/1
  Mux3/1 -> mpc_umin/1
  DataTypeConversion_extmv/1(y) -> mpc_ext_mv/1
  "Relative yaw angle reference constant "/1 -> Mux/3
  Switching controller with bumpless transfer/1 -> DataTypeConversion_extmv/1(u)
  Set velocity/1 -> DataTypeConversion_vset/1
  Minimum acceleration/1 -> DataTypeConversion_amin/1
  DataTypeConversion_umax/1 -> Mux5/2
  DataTypeConversion_Vx/1 -> Product/2, mpc_mo_Vx/1
  DataTypeConversion_amax/1 -> Mux5/1
  DataTypeConversion_umin/1 -> Mux3/2
  Lateral deviation/1 -> DataTypeConversion_e1/1
  Maximum acceleration/1 -> DataTypeConversion_amax/1
  DataTypeConversion_e2/1 -> mpc_mo_e2/1
  Product/1 -> mpc_md/1
  CurvatureConversion/1 -> Product/1
  DataTypeConversion_amin/1 -> Mux3/1
  Minimum steering angle/1 -> DataTypeConversion_umin/1
  Maximum steering angle/1 -> DataTypeConversion_umax/1
  Lateral deviation reference constant/1 -> Mux/2
  Mux5/1 -> mpc_umax/1
  Curvature/1 -> CurvatureConversion/1
  Longitudinal velocity/1 -> DataTypeConversion_Vx/1

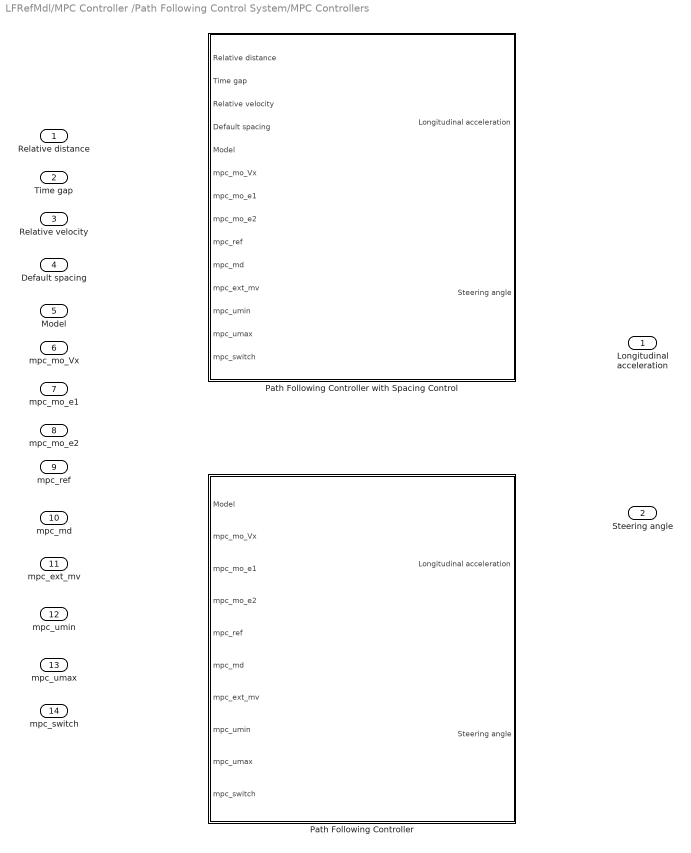
== system LFRefMdl/MPC Controller /Path Following Control System/MPC Controllers ==
  "Relative distance " : Inport
  "Time gap " : Inport  Port=2
  "Relative velocity " : Inport  Port=3
  "Default spacing " : Inport  Port=4
  "Model " : Inport  Port=5
  "mpc_mo_Vx " : Inport  Port=6
  "mpc_mo_e1 " : Inport  Port=7
  "mpc_mo_e2 " : Inport  Port=8
  "mpc_ref " : Inport  Port=9
  "mpc_md " : Inport  Port=10
  "mpc_ext_mv " : Inport  Port=11
  "mpc_umin " : Inport  Port=12
  "mpc_umax " : Inport  Port=13
  "mpc_switch " : Inport  Port=14
  Path Following Controller : Subsystem  VariantControl=pathFollowingNoSpacingCtrl
  Path Following Controller with Spacing Control : Subsystem  VariantControl=pathFollowingHasSpacingCtrl
  " Longitudinal acceleration" : Outport  VectorParamsAs1DForOutWhenUnconnected=off
  "  Steering angle" : Outport  Port=2  VectorParamsAs1DForOutWhenUnconnected=off

== system LFRefMdl/MPC Controller /Path Following Control System/MPC Models ==
  Sample time : Inport
  Transport lag : Inport  Port=2
  Ag : Inport  Port=3
  Bg : Inport  Port=4
  Cg : Inport  Port=5
  "Longitudinal velocity " : Inport  Port=6
  MPC Model : Subsystem  VariantControl=pathFollowingNoSpacingCtrl
  MPC Model with Spacing Control : Subsystem  VariantControl=pathFollowingHasSpacingCtrl
  " Model" : Outport  VectorParamsAs1DForOutWhenUnconnected=off

== system LFRefMdl/MPC Controller /Path Following Control System/Vehicle Models ==
  Vehicle dynamics matrix A : Inport
  Vehicle dynamics matrix B : Inport  Port=2
  Vehicle dynamics matrix C : Inport  Port=3
  "Vx " : Inport  Port=4
  Vehicle external model : Subsystem  VariantControl=useVehicleModel
  Vehicle parametric model : Subsystem  VariantControl=useVehicleParameters
  " A" : Outport  VectorParamsAs1DForOutWhenUnconnected=off
  " B" : Outport  Port=2  VectorParamsAs1DForOutWhenUnconnected=off
  " C" : Outport  Port=3  VectorParamsAs1DForOutWhenUnconnected=off

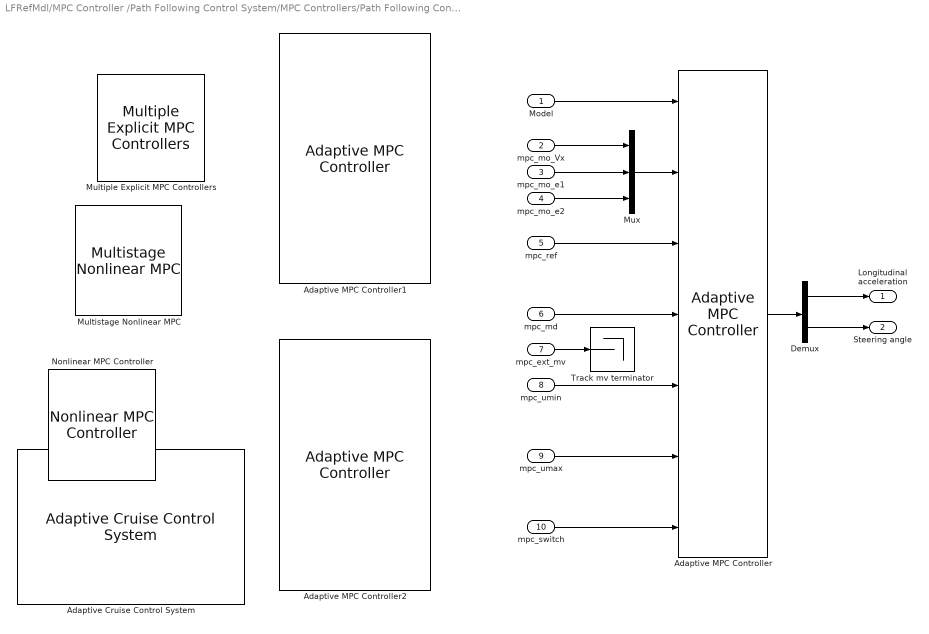
== system LFRefMdl/MPC Controller /Path Following Control System/MPC Controllers/Path Following Controller ==
  Model : Inport
  mpc_mo_Vx : Inport  Port=2
  mpc_mo_e1 : Inport  Port=3
  mpc_mo_e2 : Inport  Port=4
  mpc_ref : Inport  Port=5
  mpc_md : Inport  Port=6
  mpc_ext_mv : Inport  Port=7
  mpc_umin : Inport  Port=8
  mpc_umax : Inport  Port=9
  mpc_switch : Inport  Port=10
  Adaptive Cruise Control System : mpcadaslib/Adaptive Cruise Control System  EgoModel=tf(1,[0.5,1,0])  InitialEgoVelocity=20  DefaultSpacing=10  MaxVelocity=50  MinAcceleration=-3  amin_ext=off  MaxAcceleration=2  amax_ext=off  Ts=0.1  PredictionHorizon=30  ControllerBehavior=0.5  suboptimal=off  maxiter=10  datatypeopt=double  optmode=off  trackmode=off
  Adaptive MPC Controller : mpclib/Adaptive MPC Controller  SCDEnableBlockLinearizationSpecification=on  mpcobj=mpcobj  enable_value=0  updateMPCinCallerWorkspace=off  md_inport=on  mv_inport=off  uref_inport=off  return_cost=off  return_mvseq=off  return_qpstatus=off  return_xseq=off  return_state=off  return_ovseq=off  state_inport=off  isltv_plant=off  umin_inport=on  umax_inport=on  ymin_inport=off  ymax_inport=off  cc_inport=off  ywt_inport=off  uwt_inport=off  duwt_inport=off  rhoeps_inport=off  pm_inport=off  MaximumP=10  HorizonChoice=FixedHorizon  BlockDataType=double  SampleTimeInherited=off  switch_inport=on
  Adaptive MPC Controller1 : mpclib/Adaptive MPC Controller  SCDEnableBlockLinearizationSpecification=on  enable_value=0  updateMPCinCallerWorkspace=on  md_inport=on  mv_inport=off  uref_inport=off  return_cost=off  return_mvseq=off  return_qpstatus=off  return_xseq=off  return_state=off  return_ovseq=off  state_inport=off  isltv_plant=off  umin_inport=off  umax_inport=off  ymin_inport=off  ymax_inport=off  cc_inport=off  ywt_inport=off  uwt_inport=off  duwt_inport=off  rhoeps_inport=off  pm_inport=off  MaximumP=10  HorizonChoice=FixedHorizon  BlockDataType=double  SampleTimeInherited=off  switch_inport=off
  Adaptive MPC Controller2 : mpclib/Adaptive MPC Controller  SCDEnableBlockLinearizationSpecification=on  enable_value=0  updateMPCinCallerWorkspace=on  md_inport=on  mv_inport=on  uref_inport=off  return_cost=off  return_mvseq=off  return_qpstatus=off  return_xseq=off  return_state=off  return_ovseq=off  state_inport=off  isltv_plant=off  umin_inport=off  umax_inport=off  ymin_inport=off  ymax_inport=off  cc_inport=off  ywt_inport=off  uwt_inport=off  duwt_inport=off  rhoeps_inport=off  pm_inport=off  MaximumP=10  HorizonChoice=FixedHorizon  BlockDataType=double  SampleTimeInherited=off  switch_inport=off
  Demux : Demux  Outputs=2
  Multiple Explicit MPC Controllers : mpclib/Multiple Explicit MPC Controllers  empcobjs={''}  x0s={'[]'}  Nempc=1  theEMPC=1  nmv=1  nmo=1  nmd=1  nts=1  md_inport_multiple=on  mv_inport_multiple=off  return_status_multiple=off  return_region_multiple=off  return_state_multiple=off  state_inport_multiple=off  BlockDataType_multiple=double  SampleTimeInherited_multiple=off
  Multistage Nonlinear MPC : mpclib/Multistage Nonlinear MPC  UseObjectTs=on  UseMEX=off  md_enabled=off  stateparam_enabled=off  stageparam_enabled=off  cost_enabled=off  mvseq_enabled=off  stateseq_enabled=off  slack_enabled=off  status_enabled=off  mv_min=off  mv_max=off  mvrate_min=off  mvrate_max=off  state_min=off  state_max=off  terminal_state=off  nlp_initialize=off
  Mux : Mux  Inputs=3
  Nonlinear MPC Controller : mpclib/Nonlinear MPC Controller  UseObjectTs=on  UseMEX=off  md_enabled=off  mvtarget_enabled=off  param_enabled=off  cost_enabled=off  mvseq_enabled=off  stateseq_enabled=off  ovseq_enabled=off  slack_enabled=off  status_enabled=off  ov_min=off  ov_max=off  mv_min=off  mv_max=off  mvrate_min=off  mvrate_max=off  state_min=off  state_max=off  ov_weight=off  mv_weight=off  mvrate_weight=off  ecr_weight=off  nlp_initialize=off
  Track mv terminator : Terminator
  Longitudinal acceleration : Outport  Unit=m/s^2  VectorParamsAs1DForOutWhenUnconnected=off
  " Steering angle" : Outport  Port=2  Unit=rad  VectorParamsAs1DForOutWhenUnconnected=off
  wires:
  mpc_ext_mv/1 -> Track mv terminator/1
  Demux/2 -> " Steering angle"/1
  Demux/1 -> Longitudinal acceleration/1
  mpc_switch/1 -> Adaptive MPC Controller/7
  mpc_umin/1 -> Adaptive MPC Controller/5
  mpc_umax/1 -> Adaptive MPC Controller/6
  mpc_md/1 -> Adaptive MPC Controller/4
  mpc_ref/1 -> Adaptive MPC Controller/3
  mpc_mo_e1/1 -> Mux/2
  mpc_mo_e2/1 -> Mux/3
  Model/1 -> Adaptive MPC Controller/1
  Mux/1 -> Adaptive MPC Controller/2
  Adaptive MPC Controller/1 -> Demux/1
  mpc_mo_Vx/1 -> Mux/1

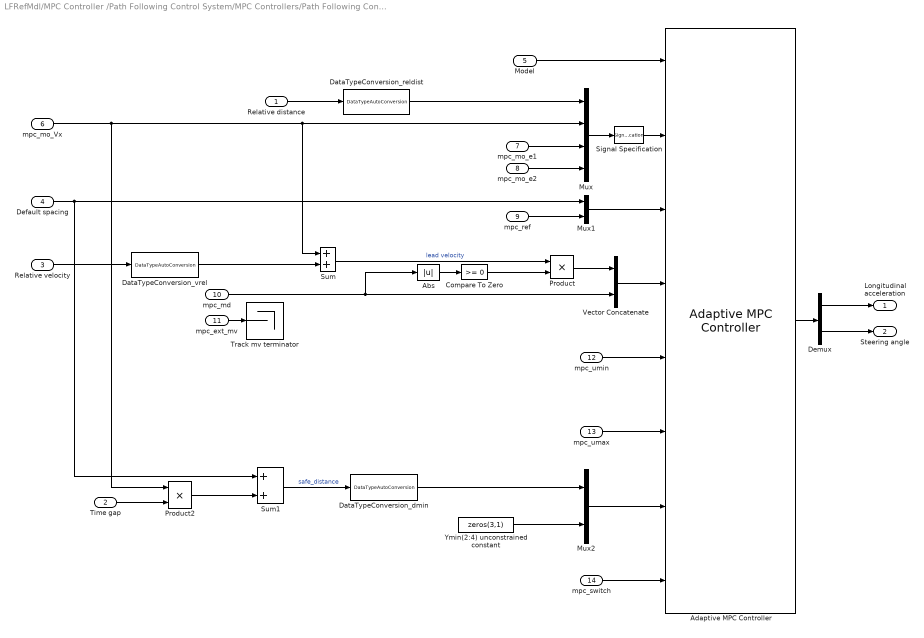
== system LFRefMdl/MPC Controller /Path Following Control System/MPC Controllers/Path Following Controller with Spacing Control ==
  Relative distance : Inport  Unit=m
  Time gap : Inport  Port=2
  Relative velocity : Inport  Port=3  Unit=m/s
  Default spacing : Inport  Port=4
  Model : Inport  Port=5
  mpc_mo_Vx : Inport  Port=6
  mpc_mo_e1 : Inport  Port=7
  mpc_mo_e2 : Inport  Port=8
  mpc_ref : Inport  Port=9
  mpc_md : Inport  Port=10
  mpc_ext_mv : Inport  Port=11
  mpc_umin : Inport  Port=12
  mpc_umax : Inport  Port=13
  mpc_switch : Inport  Port=14
  Abs : Abs  ZeroCross=off  SaturateOnIntegerOverflow=off
  Adaptive MPC Controller : mpclib/Adaptive MPC Controller  SCDEnableBlockLinearizationSpecification=on  mpcobj=mpcobj  enable_value=0  updateMPCinCallerWorkspace=off  md_inport=on  mv_inport=off  uref_inport=off  return_cost=off  return_mvseq=off  return_qpstatus=off  return_xseq=off  return_state=off  return_ovseq=off  state_inport=off  isltv_plant=off  umin_inport=on  umax_inport=on  ymin_inport=on  ymax_inport=off  cc_inport=off  ywt_inport=off  uwt_inport=off  duwt_inport=off  rhoeps_inport=off  pm_inport=off  MaximumP=10  HorizonChoice=FixedHorizon  BlockDataType=double  SampleTimeInherited=off  switch_inport=on
      link override MPC/optimizer: AllowFlexibleInterface=on
  Compare To Zero : simulink/Logic and Bit Operations/Compare To Zero  relop=>=  OutDataTypeStr=boolean  ZeroCross=off
  DataTypeConversion_dmin : mpcsigdimcheck_private/DataTypeAutoConversion  datatypestr=DataType
  DataTypeConversion_reldist : mpcsigdimcheck_private/DataTypeAutoConversion  datatypestr=DataType
  DataTypeConversion_vrel : mpcsigdimcheck_private/DataTypeAutoConversion  datatypestr=DataType
  Demux : Demux  Outputs=2
  Mux : Mux
  Mux1 : Mux  Inputs=2
  Mux2 : Mux  Inputs=2
  Product : Product
  Product2 : Product
  Signal Specification : SignalSpecification  Dimensions=4
  Sum : Sum
  Sum1 : Sum
  Track mv terminator : Terminator
  Vector Concatenate : Concatenate  Mode=Multidimensional array  ConcatenateDimension=2
  Ymin(2:4) unconstrained constant : Constant  Value=zeros(3,1)  VectorParams1D=off  OutDataTypeStr=DataType
  Longitudinal acceleration : Outport  Unit=m/s^2  VectorParamsAs1DForOutWhenUnconnected=off
  " Steering angle" : Outport  Port=2  Unit=rad  VectorParamsAs1DForOutWhenUnconnected=off
  wires:
  Product/1 -> Vector Concatenate/1
  Compare To Zero/1 -> Product/2
  mpc_md/1 -> Vector Concatenate/2, Abs/1
  Abs/1 -> Compare To Zero/1
  DataTypeConversion_vrel/1 -> Sum/2
  mpc_ext_mv/1 -> Track mv terminator/1
  mpc_ref/1 -> Mux1/2
  Vector Concatenate/1 -> Adaptive MPC Controller/4
  Signal Specification/1 -> Adaptive MPC Controller/2
  DataTypeConversion_dmin/1 -> Mux2/1
  Demux/2 -> " Steering angle"/1
  Sum/1 -> Product/1  "lead velocity"
  Sum1/1 -> DataTypeConversion_dmin/1  "safe_distance"
  Time gap/1 -> Product2/2
  mpc_mo_e1/1 -> Mux/3
  Adaptive MPC Controller/1 -> Demux/1
  mpc_switch/1 -> Adaptive MPC Controller/8
  Product2/1 -> Sum1/2
  Relative distance/1 -> DataTypeConversion_reldist/1
  Mux1/1 -> Adaptive MPC Controller/3
  mpc_umax/1 -> Adaptive MPC Controller/6
  mpc_mo_Vx/1 -> Sum/1, Mux/2, Product2/1
  Relative velocity/1 -> DataTypeConversion_vrel/1
  Default spacing/1 -> Sum1/1, Mux1/1
  Mux/1 -> Signal Specification/1
  mpc_mo_e2/1 -> Mux/4
  Model/1 -> Adaptive MPC Controller/1
  Demux/1 -> Longitudinal acceleration/1
  mpc_umin/1 -> Adaptive MPC Controller/5
  DataTypeConversion_reldist/1 -> Mux/1
  Ymin(2:4) unconstrained constant/1 -> Mux2/2
  Mux2/1 -> Adaptive MPC Controller/7
